simulink model "estimator_ekf_v02"  (Simulink 7.0)
settings: Solver=FixedStepDiscrete  StartTime=0  StopTime=0  FixedStep=1e-3  RelTol=1e-3
undefined symbols (not defined in the file): Ilf, Irf, l_fts, P0, Q, R, ROBOT, ts, X0
libraries: simulink x8
settings Model: Creator=raje_ra  LastModifiedBy=raje_ra  ExtModeAutoUpdateStatusClock=off
settings DebuggingCC: SignalInfNanChecking=error  CheckMatrixSingularityMsg=warning

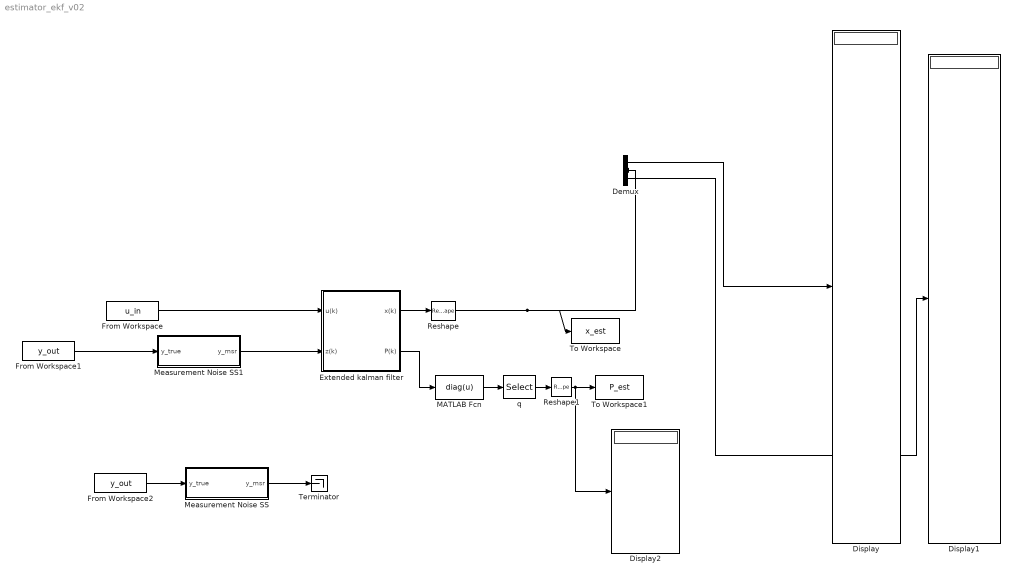
== system estimator_ekf_v02 ==
  Demux : Demux  Outputs=2
  Display : Display
  Display1 : Display
  Display2 : Display
  Extended kalman filter : Subsystem
  From Workspace : FromWorkspace  VariableName=u_in  SampleTime=0
  From Workspace1 : FromWorkspace  VariableName=y_out  SampleTime=0
  From Workspace2 : FromWorkspace  VariableName=y_out  SampleTime=0
  MATLAB Fcn : MATLABFcn  MATLABFcn=diag(u)  Output1D=off
  Measurement Noise SS : Subsystem
  Measurement Noise SS1 : Subsystem
  Reshape : Reshape
  Reshape1 : Reshape
  Terminator : Terminator
  To Workspace : ToWorkspace  VariableName=x_est  SampleTime=-1  SaveFormat=Structure With Time
  To Workspace1 : ToWorkspace  VariableName=P_est  SampleTime=-1  SaveFormat=Structure With Time
  q : Selector  InputPortWidth=62  IndexOptions=Index vector (dialog)  Indices=[1:6 32:37]  OutputSizes=1
  wires:
  Extended kalman filter/1(x(k)) -> Reshape/1
  From Workspace1/1 -> Measurement Noise SS1/1(y_true)
  From Workspace/1 -> Extended kalman filter/1(u(k))
  Reshape/1 -> To Workspace/1, Demux/1
  Measurement Noise SS/1(y_msr) -> Terminator/1
  From Workspace2/1 -> Measurement Noise SS/1(y_true)
  Measurement Noise SS1/1(y_msr) -> Extended kalman filter/2(z(k))
  Extended kalman filter/2(P(k)) -> MATLAB Fcn/1
  Demux/1 -> Display/1
  Demux/2 -> Display1/1
  MATLAB Fcn/1 -> q/1
  q/1 -> Reshape1/1
  Reshape1/1 -> To Workspace1/1, Display2/1

== system estimator_ekf_v02/Extended kalman filter ==
  u(k) : Inport  OutDataType=sfix(16)  OutScaling=2^0
  z(k) : Inport  Port=2  OutDataType=sfix(16)  OutScaling=2^0
  Unit Delay : UnitDelay  X0=X0  SampleTime=ts
  Unit Delay1 : UnitDelay  X0=P0  SampleTime=ts
  contact measurements : Subsystem
  corrector : Subsystem
  predictor : Subsystem
  x(k) : Outport  OutDataType=sfix(16)  OutScaling=2^0
  P(k) : Outport  Port=2  OutDataType=sfix(16)  OutScaling=2^0
  wires:
  u(k)/1 -> predictor/1(u(k)), corrector/2(u(k)), contact measurements/2(u_in(k))
  predictor/2(x_(k)-) -> corrector/4(x_(k)-)
  Unit Delay/1 -> predictor/2(x(k-1))
  corrector/1(x(k)) -> Unit Delay/1, x(k)/1  "x(k)"
  Unit Delay1/1 -> predictor/3(P(k-1))
  predictor/1(P_(k)-) -> corrector/3(P_(k)-)
  corrector/2(P(k)) -> Unit Delay1/1, P(k)/1
  z(k)/1 -> contact measurements/1(y(k))
  contact measurements/1(y) -> corrector/1(z(k))

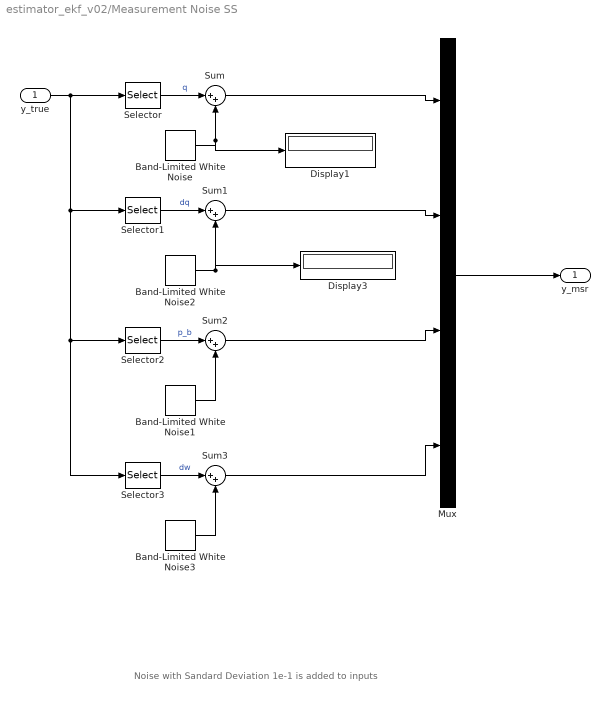
== system estimator_ekf_v02/Measurement Noise SS ==
  note: Noise with Sandard Deviation 1e-1 is added to inputs
  y_true : Inport  OutDataType=sfix(16)  OutScaling=2^0
  Band-Limited White Noise : simulink/Sources/Band-Limited White Noise  SystemSampleTime=-1  Cov=[1e-9]  Ts=ts  seed=[23341]
  Band-Limited White Noise1 : simulink/Sources/Band-Limited White Noise  SystemSampleTime=-1  Cov=[1e-8]  Ts=ts  seed=[23341]
  Band-Limited White Noise2 : simulink/Sources/Band-Limited White Noise  SystemSampleTime=-1  Cov=[1e-9]  Ts=ts  seed=[23341]
  Band-Limited White Noise3 : simulink/Sources/Band-Limited White Noise  SystemSampleTime=-1  Cov=[1e-9]  Ts=ts  seed=[23341]
  Display1 : Display
  Display3 : Display
  Mux : Mux
  Selector : Selector  InputPortWidth=m  IndexOptions=Index vector (dialog)  Indices=[1:25]  OutputSizes=1
  Selector1 : Selector  InputPortWidth=m  IndexOptions=Index vector (dialog)  Indices=[26:50]  OutputSizes=1
  Selector2 : Selector  InputPortWidth=m  IndexOptions=Index vector (dialog)  Indices=[51:53]  OutputSizes=1
  Selector3 : Selector  InputPortWidth=m  IndexOptions=Index vector (dialog)  Indices=[54:56]  OutputSizes=1
  Sum{,1..3} (4 alike) : Sum  Inputs=|++  OutDataType=sfix(16)  OutScaling=2^0
  y_msr : Outport
  wires:
  Band-Limited White Noise/1 -> Sum/2, Display1/1
  y_true/1 -> Selector/1, Selector1/1, Selector2/1, Selector3/1
  Selector/1 -> Sum/1  "q"
  Selector1/1 -> Sum1/1  "dq"
  Band-Limited White Noise2/1 -> Sum1/2, Display3/1
  Band-Limited White Noise1/1 -> Sum2/2
  Selector2/1 -> Sum2/1  "p_b"
  Band-Limited White Noise3/1 -> Sum3/2
  Selector3/1 -> Sum3/1  "dw"
  Sum/1 -> Mux/1
  Sum1/1 -> Mux/2
  Sum2/1 -> Mux/3
  Sum3/1 -> Mux/4
  Mux/1 -> y_msr/1

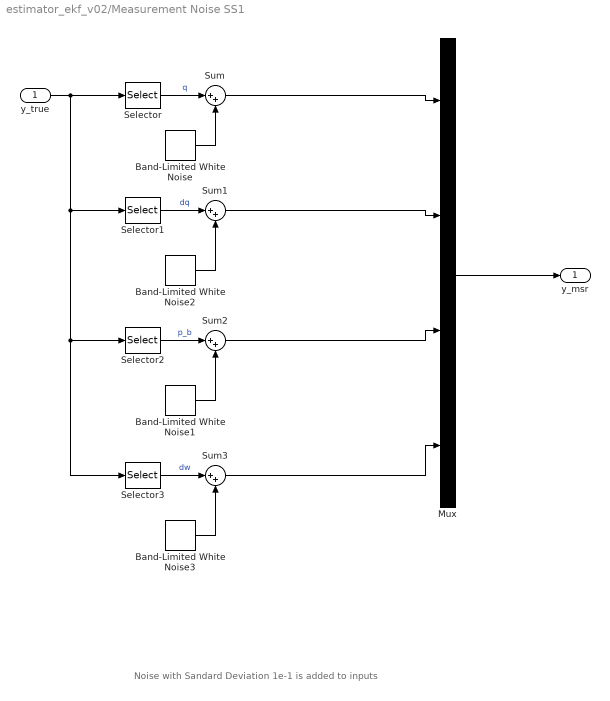
== system estimator_ekf_v02/Measurement Noise SS1 ==
  note: Noise with Sandard Deviation 1e-1 is added to inputs
  y_true : Inport  OutDataType=sfix(16)  OutScaling=2^0
  Band-Limited White Noise : simulink/Sources/Band-Limited White Noise  SystemSampleTime=-1  Cov=[1e-9]  Ts=ts  seed=[23341]
  Band-Limited White Noise1 : simulink/Sources/Band-Limited White Noise  SystemSampleTime=-1  Cov=[1e-5]  Ts=ts  seed=[23341]
  Band-Limited White Noise2 : simulink/Sources/Band-Limited White Noise  SystemSampleTime=-1  Cov=[1e-7]  Ts=ts  seed=[23341]
  Band-Limited White Noise3 : simulink/Sources/Band-Limited White Noise  SystemSampleTime=-1  Cov=[1e-7]  Ts=ts  seed=[23341]
  Mux : Mux
  Selector : Selector  InputPortWidth=m  IndexOptions=Index vector (dialog)  Indices=[1:25]  OutputSizes=1
  Selector1 : Selector  InputPortWidth=m  IndexOptions=Index vector (dialog)  Indices=[26:50]  OutputSizes=1
  Selector2 : Selector  InputPortWidth=m  IndexOptions=Index vector (dialog)  Indices=[51:53]  OutputSizes=1
  Selector3 : Selector  InputPortWidth=m  IndexOptions=Index vector (dialog)  Indices=[54:56]  OutputSizes=1
  Sum{,1..3} (4 alike) : Sum  Inputs=|++  OutDataType=sfix(16)  OutScaling=2^0
  y_msr : Outport
  wires:
  Mux/1 -> y_msr/1
  Sum3/1 -> Mux/4
  Sum2/1 -> Mux/3
  Sum1/1 -> Mux/2
  Sum/1 -> Mux/1
  Selector3/1 -> Sum3/1  "dw"
  Band-Limited White Noise3/1 -> Sum3/2
  Selector2/1 -> Sum2/1  "p_b"
  Band-Limited White Noise1/1 -> Sum2/2
  Band-Limited White Noise2/1 -> Sum1/2
  Selector1/1 -> Sum1/1  "dq"
  Selector/1 -> Sum/1  "q"
  y_true/1 -> Selector3/1, Selector2/1, Selector1/1, Selector/1
  Band-Limited White Noise/1 -> Sum/2

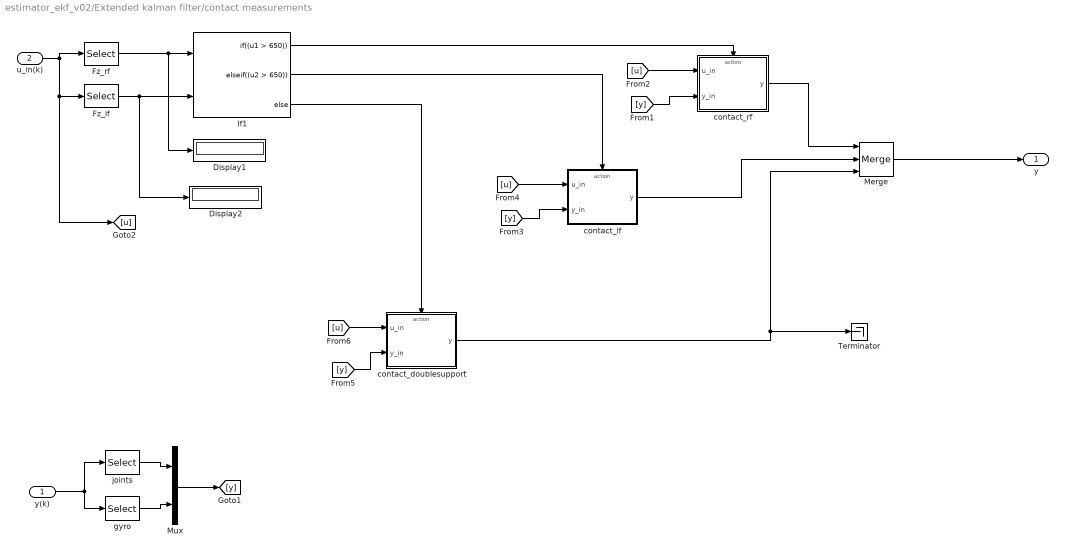
== system estimator_ekf_v02/Extended kalman filter/contact measurements ==
  y(k) : Inport
  u_in(k) : Inport  Port=2
  Display1 : Display
  Display2 : Display
  Fz_lf : Selector  InputPortWidth=37  IndexOptions=Index vector (dialog)  Indices=3  OutputSizes=1
  Fz_rf : Selector  InputPortWidth=37  IndexOptions=Index vector (dialog)  Indices=3  OutputSizes=1
  If1 : If  NumInputs=2  IfExpression=(u1 > 650)  ElseIfExpressions=(u2 > 650)
  Merge : Merge  Inputs=3
  Mux : Mux  Inputs=2
  Terminator : Terminator
  contact_doublesupport : Subsystem
  contact_lf : Subsystem
  contact_rf : Subsystem
  gyro : Selector  InputPortWidth=56  IndexOptions=Index vector (dialog)  Indices=[51:56]  OutputSizes=1
  joints : Selector  InputPortWidth=56  IndexOptions=Index vector (dialog)  Indices=1:50  OutputSizes=1
  y : Outport
  wires:
  Mux/1 -> [y]
  gyro/1 -> Mux/2
  joints/1 -> Mux/1
  contact_doublesupport/1(y) -> Merge/3, Terminator/1
  Merge/1 -> y/1
  contact_lf/1(y) -> Merge/2
  contact_rf/1(y) -> Merge/1
  If1/3 -> contact_doublesupport/Action
  If1/2 -> contact_lf/Action
  [y] -> contact_doublesupport/2(y_in)
  [u] -> contact_doublesupport/1(u_in)
  [y] -> contact_lf/2(y_in)
  [u] -> contact_lf/1(u_in)
  [y] -> contact_rf/2(y_in)
  [u] -> contact_rf/1(u_in)
  If1/1 -> contact_rf/Action
  u_in(k)/1 -> [u], Fz_lf/1, Fz_rf/1
  Fz_lf/1 -> Display2/1, If1/2
  Fz_rf/1 -> Display1/1, If1/1
  y(k)/1 -> gyro/1, joints/1

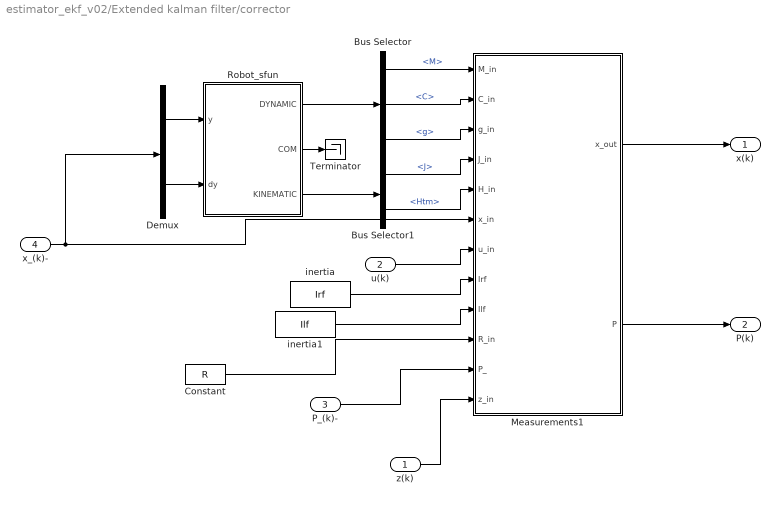
== system estimator_ekf_v02/Extended kalman filter/corrector ==
  z(k) : Inport  OutDataType=sfix(16)  OutScaling=2^0
  u(k) : Inport  Port=2  OutDataType=sfix(16)  OutScaling=2^0
  P_(k)- : Inport  Port=3  OutDataType=sfix(16)  OutScaling=2^0
  x_(k)- : Inport  Port=4  OutDataType=sfix(16)  OutScaling=2^0
  Bus Selector : BusSelector  OutputSignals=M,C,g
  Bus Selector1 : BusSelector  OutputSignals=J,Htm
  Constant : Constant  Value=R  OutDataType=sfix(16)  OutScaling=2^0
  Demux : Demux  Outputs=2
  Measurements1 : Stateflow chart
  Robot_sfun : Subsystem
  Terminator : Terminator
  inertia : Constant  Value=Irf  VectorParams1D=off  OutDataType=sfix(16)  OutScaling=2^0
  inertia1 : Constant  Value=Ilf  VectorParams1D=off  OutDataType=sfix(16)  OutScaling=2^0
  x(k) : Outport  OutDataType=sfix(16)  OutScaling=2^0
  P(k) : Outport  Port=2  OutDataType=sfix(16)  OutScaling=2^0
  wires:
  Robot_sfun/1(DYNAMIC) -> Bus Selector/1
  Bus Selector/1 -> Measurements1/1(M_in)  "<M>"
  Bus Selector/2 -> Measurements1/2(C_in)  "<C>"
  Bus Selector/3 -> Measurements1/3(g_in)  "<g>"
  Robot_sfun/3(KINEMATIC) -> Bus Selector1/1
  Bus Selector1/1 -> Measurements1/4(J_in)  "<J>"
  Bus Selector1/2 -> Measurements1/5(H_in)  "<Htm>"
  Demux/1 -> Robot_sfun/1(y)
  Demux/2 -> Robot_sfun/2(dy)
  Robot_sfun/2(COM) -> Terminator/1
  x_(k)-/1 -> Demux/1, Measurements1/6(x_in)
  Measurements1/1(x_out) -> x(k)/1
  u(k)/1 -> Measurements1/7(u_in)
  inertia/1 -> Measurements1/8(Irf)
  inertia1/1 -> Measurements1/9(Ilf)
  Constant/1 -> Measurements1/10(R_in)
  P_(k)-/1 -> Measurements1/11(P_)
  Measurements1/2(P) -> P(k)/1
  z(k)/1 -> Measurements1/12(z_in)

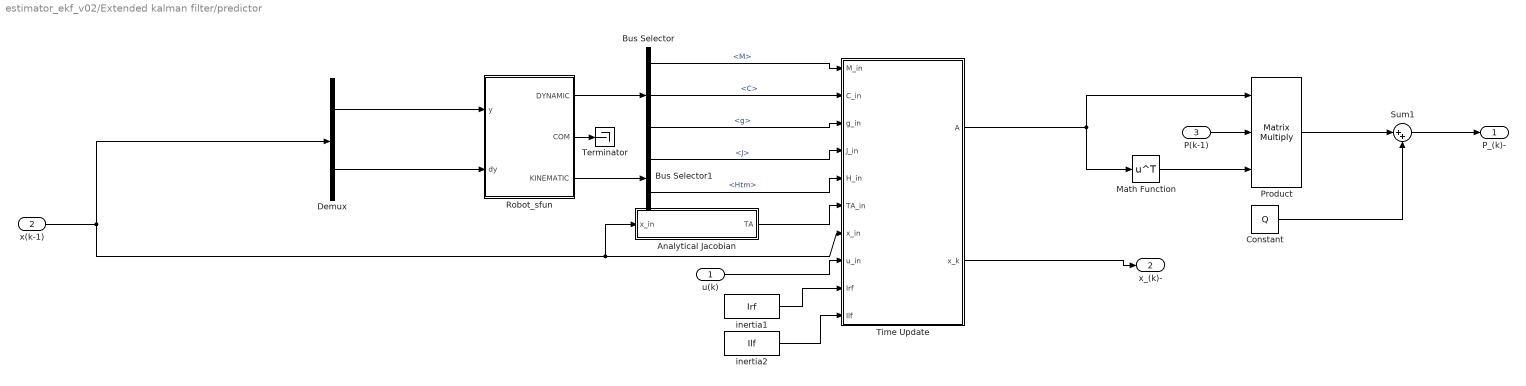
== system estimator_ekf_v02/Extended kalman filter/predictor ==
  u(k) : Inport  OutDataType=sfix(16)  OutScaling=2^0
  x(k-1) : Inport  Port=2  OutDataType=sfix(16)  OutScaling=2^0
  P(k-1) : Inport  Port=3  OutDataType=sfix(16)  OutScaling=2^0
  Analytical Jacobian : Stateflow chart
  Bus Selector : BusSelector  OutputSignals=M,C,g
  Bus Selector1 : BusSelector  OutputSignals=J,Htm
  Constant : Constant  Value=Q  OutDataType=sfix(16)  OutScaling=2^0
  Demux : Demux  Outputs=2
  Math Function : Math  Operator=transpose  OutDataType=sfix(16)  OutScaling=2^0  SaturateOnIntegerOverflow=on
  Product : Product  Inputs=3  Multiplication=Matrix(*)  OutDataType=sfix(16)  OutScaling=2^0  RndMeth=Zero
  Robot_sfun : Subsystem
  Sum1 : Sum  Inputs=|++  OutDataType=sfix(16)  OutScaling=2^0
  Terminator : Terminator
  Time Update : Stateflow chart
  inertia1 : Constant  Value=Irf  VectorParams1D=off  OutDataType=sfix(16)  OutScaling=2^0
  inertia2 : Constant  Value=Ilf  VectorParams1D=off  OutDataType=sfix(16)  OutScaling=2^0
  P_(k)- : Outport  OutDataType=sfix(16)  OutScaling=2^0
  x_(k)- : Outport  Port=2  OutDataType=sfix(16)  OutScaling=2^0
  wires:
  Robot_sfun/1(DYNAMIC) -> Bus Selector/1
  Bus Selector/1 -> Time Update/1(M_in)  "<M>"
  Bus Selector/2 -> Time Update/2(C_in)  "<C>"
  Bus Selector/3 -> Time Update/3(g_in)  "<g>"
  Robot_sfun/3(KINEMATIC) -> Bus Selector1/1
  Bus Selector1/1 -> Time Update/4(J_in)  "<J>"
  Bus Selector1/2 -> Time Update/5(H_in)  "<Htm>"
  x(k-1)/1 -> Analytical Jacobian/1(x_in), Time Update/7(x_in), Demux/1
  Demux/1 -> Robot_sfun/1(y)
  Demux/2 -> Robot_sfun/2(dy)
  Time Update/1(A) -> Math Function/1, Product/1
  Math Function/1 -> Product/3
  P(k-1)/1 -> Product/2
  Product/1 -> Sum1/1
  Constant/1 -> Sum1/2
  Sum1/1 -> P_(k)-/1
  Robot_sfun/2(COM) -> Terminator/1
  Analytical Jacobian/1(TA) -> Time Update/6(TA_in)
  u(k)/1 -> Time Update/8(u_in)
  inertia1/1 -> Time Update/9(Irf)
  inertia2/1 -> Time Update/10(Ilf)
  Time Update/2(x_k) -> x_(k)-/1

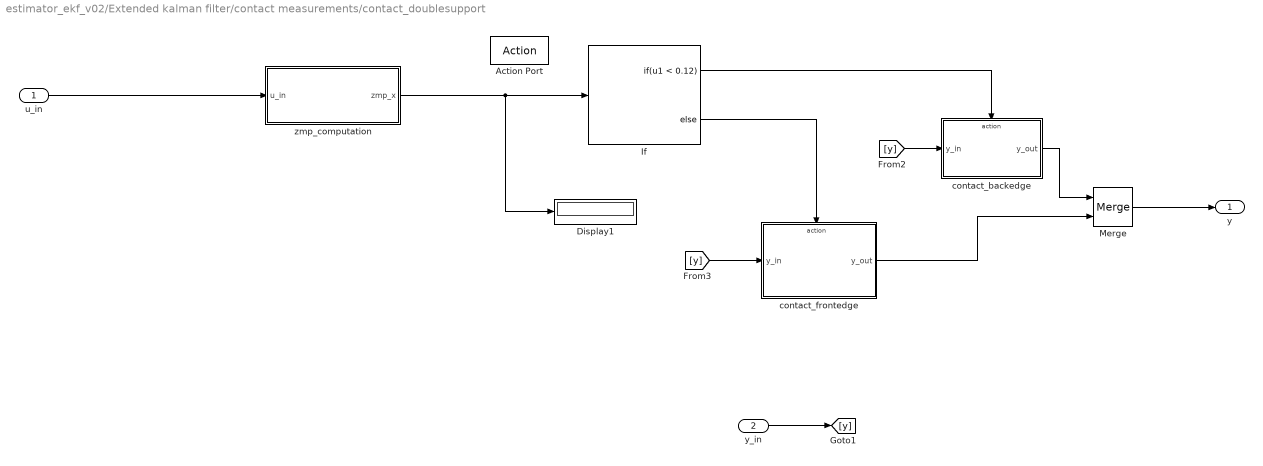
== system estimator_ekf_v02/Extended kalman filter/contact measurements/contact_doublesupport ==
  u_in : Inport
  y_in : Inport  Port=2
  Action Port : ActionPort  ActionType=else
  Display1 : Display
  If : If  IfExpression=u1 < 0.12
  Merge : Merge
  contact_backedge : Subsystem  TreatAsAtomicUnit=on
  contact_frontedge : Subsystem  TreatAsAtomicUnit=on
  zmp_computation : Subsystem
  y : Outport
  wires:
  u_in/1 -> zmp_computation/1(u_in)
  zmp_computation/1(zmp_x) -> Display1/1, If/1
  y_in/1 -> [y]
  Merge/1 -> y/1
  contact_frontedge/1(y_out) -> Merge/2
  contact_backedge/1(y_out) -> Merge/1
  [y] -> contact_frontedge/1(y_in)
  [y] -> contact_backedge/1(y_in)
  If/2 -> contact_frontedge/Action
  If/1 -> contact_backedge/Action

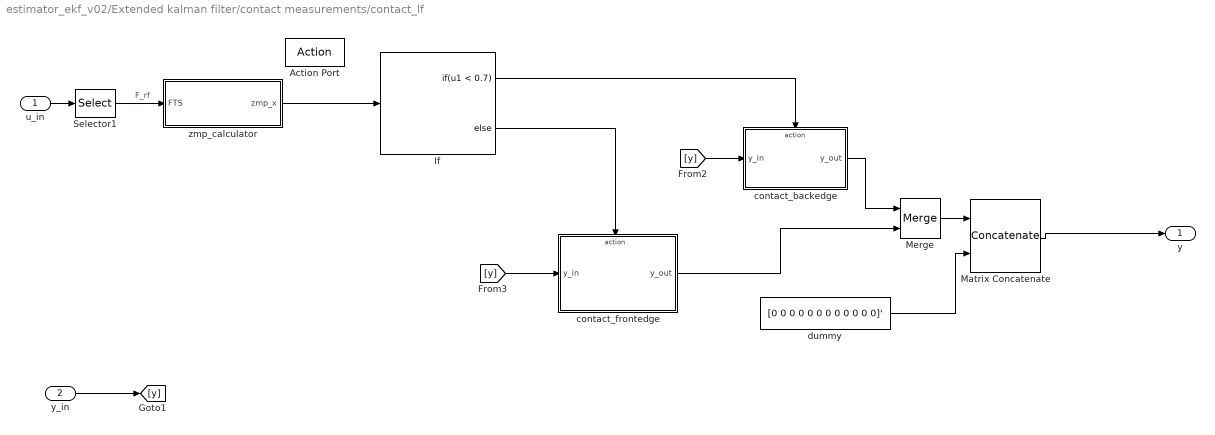
== system estimator_ekf_v02/Extended kalman filter/contact measurements/contact_lf ==
  u_in : Inport
  y_in : Inport  Port=2
  Action Port : ActionPort  ActionType=elseif
  If : If  IfExpression=u1 < 0.7
  Matrix Concatenate : Concatenate  Mode=Multidimensional array
  Merge : Merge
  Selector1 : Selector  InputPortWidth=37  IndexOptions=Index vector (dialog)  Indices=7:12  OutputSizes=1
  contact_backedge : Subsystem  TreatAsAtomicUnit=on
  contact_frontedge : Subsystem  TreatAsAtomicUnit=on
  dummy : Constant  Value=[0 0 0 0 0 0 0 0 0 0 0 0]'  VectorParams1D=off  OutDataType=sfix(16)  OutScaling=2^0
  zmp_calculator : Subsystem
  y : Outport
  wires:
  Matrix Concatenate/1 -> y/1
  dummy/1 -> Matrix Concatenate/2
  Merge/1 -> Matrix Concatenate/1
  If/1 -> contact_backedge/Action
  If/2 -> contact_frontedge/Action
  [y] -> contact_backedge/1(y_in)
  [y] -> contact_frontedge/1(y_in)
  contact_backedge/1(y_out) -> Merge/1
  contact_frontedge/1(y_out) -> Merge/2
  zmp_calculator/1(zmp_x) -> If/1
  Selector1/1 -> zmp_calculator/1(FTS)  "F_rf"
  u_in/1 -> Selector1/1
  y_in/1 -> [y]

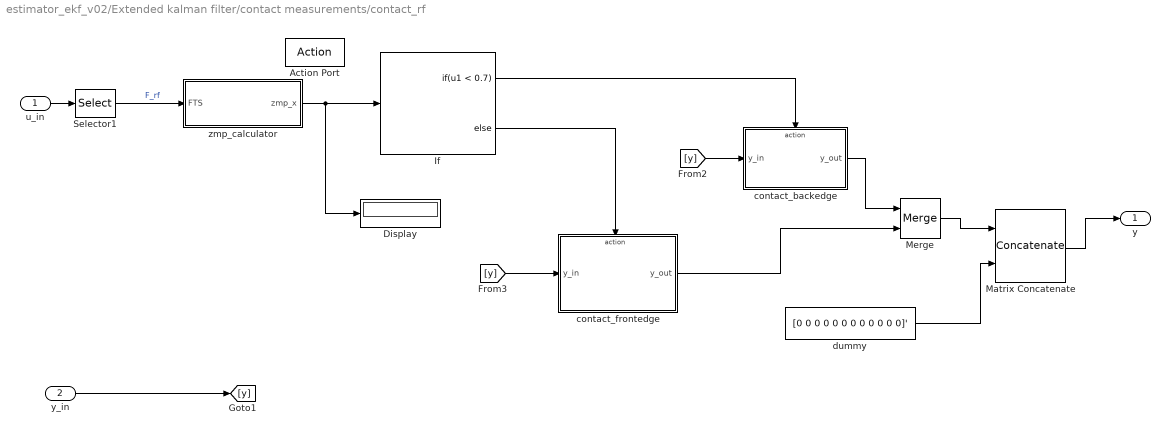
== system estimator_ekf_v02/Extended kalman filter/contact measurements/contact_rf ==
  u_in : Inport
  y_in : Inport  Port=2
  Action Port : ActionPort  ActionType=then
  Display : Display
  If : If  IfExpression=u1 < 0.7
  Matrix Concatenate : Concatenate  Mode=Multidimensional array
  Merge : Merge
  Selector1 : Selector  InputPortWidth=37  IndexOptions=Index vector (dialog)  Indices=1:6  OutputSizes=1
  contact_backedge : Subsystem  TreatAsAtomicUnit=on
  contact_frontedge : Subsystem  TreatAsAtomicUnit=on
  dummy : Constant  Value=[0 0 0 0 0 0 0 0 0 0 0 0]'  VectorParams1D=off  OutDataType=sfix(16)  OutScaling=2^0
  zmp_calculator : Subsystem
  y : Outport
  wires:
  Matrix Concatenate/1 -> y/1
  Merge/1 -> Matrix Concatenate/1
  dummy/1 -> Matrix Concatenate/2
  y_in/1 -> [y]
  u_in/1 -> Selector1/1
  Selector1/1 -> zmp_calculator/1(FTS)  "F_rf"
  zmp_calculator/1(zmp_x) -> Display/1, If/1
  contact_frontedge/1(y_out) -> Merge/2
  contact_backedge/1(y_out) -> Merge/1
  [y] -> contact_frontedge/1(y_in)
  [y] -> contact_backedge/1(y_in)
  If/2 -> contact_frontedge/Action
  If/1 -> contact_backedge/Action

== system estimator_ekf_v02/Extended kalman filter/corrector/Robot_sfun ==
  y : Inport
  dy : Inport  Port=2
  Bus Creator : BusCreator
  Bus Creator1 : BusCreator  Inputs=3
  Bus Creator2 : BusCreator  Inputs=3
  S-Function : S-Function  FunctionName=luca_dynamics_dy_sfun  Parameters=(size(ROBOT.csi,1)/6-1), size(ROBOT.csi,2), ROBOT.parent, ROBOT.tcp, ROBOT.g0, ROBOT.csi, ROBOT.com, ROBOT.Mass
  DYNAMIC : Outport
  COM : Outport  Port=2
  KINEMATIC : Outport  Port=3
  wires:
  y/1 -> S-Function/1
  dy/1 -> S-Function/2
  S-Function/1 -> Bus Creator/1  "M"
  S-Function/2 -> Bus Creator/2  "C"
  S-Function/3 -> Bus Creator/3  "g"
  S-Function/4 -> Bus Creator/4  "dM"
  S-Function/5 -> Bus Creator1/1  "x"
  S-Function/6 -> Bus Creator1/2  "J"
  S-Function/7 -> Bus Creator1/3  "dJ"
  S-Function/8 -> Bus Creator2/1  "Htm"
  S-Function/9 -> Bus Creator2/2  "J"
  S-Function/10 -> Bus Creator2/3  "dJ"
  Bus Creator/1 -> DYNAMIC/1
  Bus Creator1/1 -> COM/1
  Bus Creator2/1 -> KINEMATIC/1

== system estimator_ekf_v02/Extended kalman filter/predictor/Robot_sfun ==
  y : Inport
  dy : Inport  Port=2
  Bus Creator : BusCreator
  Bus Creator1 : BusCreator  Inputs=3
  Bus Creator2 : BusCreator  Inputs=3
  S-Function : S-Function  FunctionName=luca_dynamics_dy_sfun  Parameters=(size(ROBOT.csi,1)/6-1), size(ROBOT.csi,2), ROBOT.parent, ROBOT.tcp, ROBOT.g0, ROBOT.csi, ROBOT.com, ROBOT.Mass
  DYNAMIC : Outport
  COM : Outport  Port=2
  KINEMATIC : Outport  Port=3
  wires:
  Bus Creator2/1 -> KINEMATIC/1
  Bus Creator1/1 -> COM/1
  Bus Creator/1 -> DYNAMIC/1
  S-Function/10 -> Bus Creator2/3  "dJ"
  S-Function/9 -> Bus Creator2/2  "J"
  S-Function/8 -> Bus Creator2/1  "Htm"
  S-Function/7 -> Bus Creator1/3  "dJ"
  S-Function/6 -> Bus Creator1/2  "J"
  S-Function/5 -> Bus Creator1/1  "x"
  S-Function/4 -> Bus Creator/4  "dM"
  S-Function/3 -> Bus Creator/3  "g"
  S-Function/2 -> Bus Creator/2  "C"
  S-Function/1 -> Bus Creator/1  "M"
  dy/1 -> S-Function/2
  y/1 -> S-Function/1

== system estimator_ekf_v02/Extended kalman filter/contact measurements/contact_doublesupport/contact_backedge ==
  y_in : Inport  OutDataType=sfix(16)  OutScaling=2^0
  Action Port : ActionPort  ActionType=then
  Matrix Concatenate : Concatenate  NumInputs=4  Mode=Multidimensional array
  V_feet : Constant  Value=[0 0 0 0 0 0 0 0 0 0 0 0]'  VectorParams1D=off  OutDataType=sfix(16)  OutScaling=2^0
  lf_contact_CD : Constant  Value="[-0.059999942250943   0.065450013201346  -0.000099999469068  -0.059999926220207   0.160450013201344  -0.000099995026751]'"  VectorParams1D=off  OutDataType=sfix(16)  OutScaling=2^0
  rf_contact_CD : Constant  Value="[-0.059999991262275  -0.160449976611997  -0.000099795625568  -0.059999972932080  -0.065449976612284  -0.000099562918613]'"  VectorParams1D=off  OutDataType=sfix(16)  OutScaling=2^0
  y_out : Outport  OutDataType=sfix(16)  OutScaling=2^0
  wires:
  V_feet/1 -> Matrix Concatenate/4
  lf_contact_CD/1 -> Matrix Concatenate/3
  rf_contact_CD/1 -> Matrix Concatenate/2
  Matrix Concatenate/1 -> y_out/1
  y_in/1 -> Matrix Concatenate/1

== system estimator_ekf_v02/Extended kalman filter/contact measurements/contact_doublesupport/contact_frontedge ==
  y_in : Inport  OutDataType=sfix(16)  OutScaling=2^0
  Action Port : ActionPort  ActionType=else
  Matrix Concatenate : Concatenate  NumInputs=4  Mode=Multidimensional array
  V_feet : Constant  Value=[0 0 0 0 0 0 0 0 0 0 0 0]'  VectorParams1D=off  OutDataType=sfix(16)  OutScaling=2^0
  lf_contact_AB : Constant  Value="[0.130000073779718   0.160449981139864  -0.000099828958185   0.130000057748982   0.065449981139865  -0.000099833400502]'"  VectorParams1D=off  OutDataType=sfix(16)  OutScaling=2^0
  rf_contact_AB : Constant  Value="[0.130000027067808  -0.065450013272176  -0.000099766533171   0.130000008737612  -0.160450013271890  -0.000099999240125]'"  VectorParams1D=off  OutDataType=sfix(16)  OutScaling=2^0
  y_out : Outport  OutDataType=sfix(16)  OutScaling=2^0
  wires:
  V_feet/1 -> Matrix Concatenate/4
  lf_contact_AB/1 -> Matrix Concatenate/3
  rf_contact_AB/1 -> Matrix Concatenate/2
  Matrix Concatenate/1 -> y_out/1
  y_in/1 -> Matrix Concatenate/1

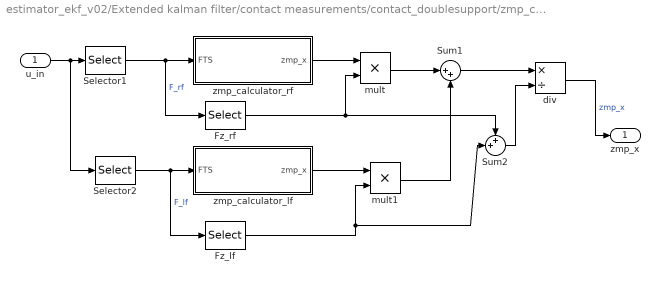
== system estimator_ekf_v02/Extended kalman filter/contact measurements/contact_doublesupport/zmp_computation ==
  u_in : Inport
  Fz_lf : Selector  InputPortWidth=6  IndexOptions=Index vector (dialog)  Indices=3  OutputSizes=1
  Fz_rf : Selector  InputPortWidth=6  IndexOptions=Index vector (dialog)  Indices=3  OutputSizes=1
  Selector1 : Selector  InputPortWidth=37  IndexOptions=Index vector (dialog)  Indices=1:6  OutputSizes=1
  Selector2 : Selector  InputPortWidth=37  IndexOptions=Index vector (dialog)  Indices=7:12  OutputSizes=1
  Sum1 : Sum  Inputs=|++  OutDataType=sfix(16)  OutScaling=2^0
  Sum2 : Sum  Inputs=++|  OutDataType=sfix(16)  OutScaling=2^0
  div : Product  Inputs=*/  OutDataType=sfix(16)  OutScaling=2^-10
  mult : Product  Inputs=**  OutDataType=sfix(16)  OutScaling=2^-10
  mult1 : Product  Inputs=**  OutDataType=sfix(16)  OutScaling=2^-10
  zmp_calculator_lf : Subsystem
  zmp_calculator_rf : Subsystem
  zmp_x : Outport
  wires:
  div/1 -> zmp_x/1  "zmp_x"
  Sum2/1 -> div/2
  Sum1/1 -> div/1
  mult1/1 -> Sum1/2
  zmp_calculator_lf/1(zmp_x) -> mult1/1
  mult/1 -> Sum1/1
  zmp_calculator_rf/1(zmp_x) -> mult/1
  Fz_rf/1 -> Sum2/1, mult/2
  Fz_lf/1 -> Sum2/2, mult1/2
  Selector2/1 -> Fz_lf/1, zmp_calculator_lf/1(FTS)  "F_lf"
  u_in/1 -> Selector2/1, Selector1/1
  Selector1/1 -> Fz_rf/1, zmp_calculator_rf/1(FTS)  "F_rf"

== system estimator_ekf_v02/Extended kalman filter/contact measurements/contact_lf/contact_backedge ==
  y_in : Inport  OutDataType=sfix(16)  OutScaling=2^0
  Action Port : ActionPort  ActionType=then
  Matrix Concatenate : Concatenate  NumInputs=3  Mode=Multidimensional array
  V_lf : Constant  Value=[0 0 0 0 0 0]'  VectorParams1D=off  OutDataType=sfix(16)  OutScaling=2^0
  lf_contact_CD : Constant  Value="[-0.059999942250943   0.065450013201346  -0.000099999469068  -0.059999926220207   0.160450013201344  -0.000099995026751]'"  VectorParams1D=off  OutDataType=sfix(16)  OutScaling=2^0
  y_out : Outport  OutDataType=sfix(16)  OutScaling=2^0
  wires:
  lf_contact_CD/1 -> Matrix Concatenate/2
  y_in/1 -> Matrix Concatenate/1
  Matrix Concatenate/1 -> y_out/1
  V_lf/1 -> Matrix Concatenate/3

== system estimator_ekf_v02/Extended kalman filter/contact measurements/contact_lf/contact_frontedge ==
  y_in : Inport  OutDataType=sfix(16)  OutScaling=2^0
  Action Port : ActionPort  ActionType=else
  Matrix Concatenate : Concatenate  NumInputs=3  Mode=Multidimensional array
  V_lf : Constant  Value=[0 0 0 0 0 0]'  VectorParams1D=off  OutDataType=sfix(16)  OutScaling=2^0
  lf_contact_AB : Constant  Value="[0.130000073779718   0.160449981139864  -0.000099828958185   0.130000057748982   0.065449981139865  -0.000099833400502]'"  VectorParams1D=off  OutDataType=sfix(16)  OutScaling=2^0
  y_out : Outport  OutDataType=sfix(16)  OutScaling=2^0
  wires:
  V_lf/1 -> Matrix Concatenate/3
  lf_contact_AB/1 -> Matrix Concatenate/2
  y_in/1 -> Matrix Concatenate/1
  Matrix Concatenate/1 -> y_out/1

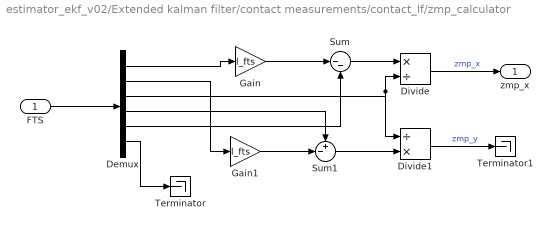
== system estimator_ekf_v02/Extended kalman filter/contact measurements/contact_lf/zmp_calculator ==
  FTS : Inport
  Demux : Demux  Outputs=6
  Divide : Product  Inputs=*/  OutDataType=sfix(16)  OutScaling=2^-10
  Divide1 : Product  Inputs=/*  OutDataType=sfix(16)  OutScaling=2^-10
  Gain : Gain  Gain=l_fts  ParameterDataType=sfix(16)  ParameterScaling=2^0  OutDataType=sfix(16)  OutScaling=2^0
  Gain1 : Gain  Gain=l_fts  ParameterDataType=sfix(16)  ParameterScaling=2^0  OutDataType=sfix(16)  OutScaling=2^0
  Sum : Sum  Inputs=|--  OutDataType=sfix(16)  OutScaling=2^0
  Sum1 : Sum  Inputs=+-|  OutDataType=sfix(16)  OutScaling=2^0
  Terminator : Terminator
  Terminator1 : Terminator
  zmp_x : Outport
  wires:
  Demux/1 -> Gain/1
  Gain/1 -> Sum/1
  Demux/5 -> Sum/2
  Sum/1 -> Divide/1
  Demux/3 -> Divide/2, Divide1/1
  Demux/2 -> Gain1/1
  Gain1/1 -> Sum1/2
  Demux/4 -> Sum1/1
  Sum1/1 -> Divide1/2
  Demux/6 -> Terminator/1
  Divide1/1 -> Terminator1/1  "zmp_y"
  Divide/1 -> zmp_x/1  "zmp_x"
  FTS/1 -> Demux/1

== system estimator_ekf_v02/Extended kalman filter/contact measurements/contact_rf/contact_backedge ==
  y_in : Inport  OutDataType=sfix(16)  OutScaling=2^0
  Action Port : ActionPort  ActionType=then
  Matrix Concatenate : Concatenate  NumInputs=3  Mode=Multidimensional array
  V_rf : Constant  Value=[0 0 0 0 0 0]'  VectorParams1D=off  OutDataType=sfix(16)  OutScaling=2^0
  rf_contact_CD : Constant  Value="[-0.059999991262275  -0.160449976611997  -0.000099795625568  -0.059999972932080  -0.065449976612284  -0.000099562918613]'"  VectorParams1D=off  OutDataType=sfix(16)  OutScaling=2^0
  y_out : Outport  OutDataType=sfix(16)  OutScaling=2^0
  wires:
  V_rf/1 -> Matrix Concatenate/3
  rf_contact_CD/1 -> Matrix Concatenate/2
  Matrix Concatenate/1 -> y_out/1
  y_in/1 -> Matrix Concatenate/1

== system estimator_ekf_v02/Extended kalman filter/contact measurements/contact_rf/contact_frontedge ==
  y_in : Inport  OutDataType=sfix(16)  OutScaling=2^0
  Action Port : ActionPort  ActionType=else
  Matrix Concatenate : Concatenate  NumInputs=3  Mode=Multidimensional array
  V_rf : Constant  Value=[0 0 0 0 0 0]'  VectorParams1D=off  OutDataType=sfix(16)  OutScaling=2^0
  rf_contact_AB : Constant  Value="[0.130000027067808  -0.065450013272176  -0.000099766533171   0.130000008737612  -0.160450013271890  -0.000099999240125]'"  VectorParams1D=off  OutDataType=sfix(16)  OutScaling=2^0
  y_out : Outport  OutDataType=sfix(16)  OutScaling=2^0
  wires:
  V_rf/1 -> Matrix Concatenate/3
  rf_contact_AB/1 -> Matrix Concatenate/2
  Matrix Concatenate/1 -> y_out/1
  y_in/1 -> Matrix Concatenate/1

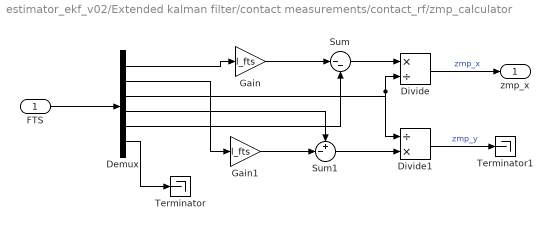
== system estimator_ekf_v02/Extended kalman filter/contact measurements/contact_rf/zmp_calculator ==
  FTS : Inport
  Demux : Demux  Outputs=6
  Divide : Product  Inputs=*/  OutDataType=sfix(16)  OutScaling=2^-10
  Divide1 : Product  Inputs=/*  OutDataType=sfix(16)  OutScaling=2^-10
  Gain : Gain  Gain=l_fts  ParameterDataType=sfix(16)  ParameterScaling=2^0  OutDataType=sfix(16)  OutScaling=2^0
  Gain1 : Gain  Gain=l_fts  ParameterDataType=sfix(16)  ParameterScaling=2^0  OutDataType=sfix(16)  OutScaling=2^0
  Sum : Sum  Inputs=|--  OutDataType=sfix(16)  OutScaling=2^0
  Sum1 : Sum  Inputs=+-|  OutDataType=sfix(16)  OutScaling=2^0
  Terminator : Terminator
  Terminator1 : Terminator
  zmp_x : Outport
  wires:
  FTS/1 -> Demux/1
  Divide/1 -> zmp_x/1  "zmp_x"
  Divide1/1 -> Terminator1/1  "zmp_y"
  Demux/6 -> Terminator/1
  Sum1/1 -> Divide1/2
  Demux/4 -> Sum1/1
  Gain1/1 -> Sum1/2
  Demux/2 -> Gain1/1
  Demux/3 -> Divide1/1, Divide/2
  Sum/1 -> Divide/1
  Demux/5 -> Sum/2
  Gain/1 -> Sum/1
  Demux/1 -> Gain/1

== system estimator_ekf_v02/Extended kalman filter/contact measurements/contact_doublesupport/zmp_computation/zmp_calculator_lf ==
  FTS : Inport
  Demux : Demux  Outputs=6
  Divide : Product  Inputs=*/  OutDataType=sfix(16)  OutScaling=2^-10
  Divide1 : Product  Inputs=/*  OutDataType=sfix(16)  OutScaling=2^-10
  Gain : Gain  Gain=l_fts  ParameterDataType=sfix(16)  ParameterScaling=2^0  OutDataType=sfix(16)  OutScaling=2^0
  Gain1 : Gain  Gain=l_fts  ParameterDataType=sfix(16)  ParameterScaling=2^0  OutDataType=sfix(16)  OutScaling=2^0
  Sum : Sum  Inputs=|--  OutDataType=sfix(16)  OutScaling=2^0
  Sum1 : Sum  Inputs=+-|  OutDataType=sfix(16)  OutScaling=2^0
  Terminator : Terminator
  Terminator1 : Terminator
  zmp_x : Outport
  wires:
  Demux/1 -> Gain/1
  Gain/1 -> Sum/1
  Demux/5 -> Sum/2
  Sum/1 -> Divide/1
  Demux/3 -> Divide/2, Divide1/1
  Demux/2 -> Gain1/1
  Gain1/1 -> Sum1/2
  Demux/4 -> Sum1/1
  Sum1/1 -> Divide1/2
  Demux/6 -> Terminator/1
  Divide1/1 -> Terminator1/1  "zmp_y"
  Divide/1 -> zmp_x/1  "zmp_x"
  FTS/1 -> Demux/1

== system estimator_ekf_v02/Extended kalman filter/contact measurements/contact_doublesupport/zmp_computation/zmp_calculator_rf ==
  FTS : Inport
  Demux : Demux  Outputs=6
  Divide : Product  Inputs=*/  OutDataType=sfix(16)  OutScaling=2^-10
  Divide1 : Product  Inputs=/*  OutDataType=sfix(16)  OutScaling=2^-10
  Gain : Gain  Gain=l_fts  ParameterDataType=sfix(16)  ParameterScaling=2^0  OutDataType=sfix(16)  OutScaling=2^0
  Gain1 : Gain  Gain=l_fts  ParameterDataType=sfix(16)  ParameterScaling=2^0  OutDataType=sfix(16)  OutScaling=2^0
  Sum : Sum  Inputs=|--  OutDataType=sfix(16)  OutScaling=2^0
  Sum1 : Sum  Inputs=+-|  OutDataType=sfix(16)  OutScaling=2^0
  Terminator : Terminator
  Terminator1 : Terminator
  zmp_x : Outport
  wires:
  FTS/1 -> Demux/1
  Divide/1 -> zmp_x/1  "zmp_x"
  Divide1/1 -> Terminator1/1  "zmp_y"
  Demux/6 -> Terminator/1
  Sum1/1 -> Divide1/2
  Demux/4 -> Sum1/1
  Gain1/1 -> Sum1/2
  Demux/2 -> Gain1/1
  Demux/3 -> Divide1/1, Divide/2
  Sum/1 -> Divide/1
  Demux/5 -> Sum/2
  Gain/1 -> Sum/1
  Demux/1 -> Gain/1

== matlab function Extended kalman filter/predictor/Analytical Jacobian ==
  data: TA output inherited; x_in input inherited
function TA = fcn(x_in)
% This block supports the Embedded MATLAB subset.
% See the help menu for details. 
% state - [ position ; velocity ]
% x_in  - [   1:31   ;   32:62  ]
ox = x_in(4);
oy = x_in(5);
% Transformation for Angular velocities to angular rates of floating base 
% on instantaneous frame of reference. x-y-z rotations.
%%{
T = [1      0           sin(oy);...
     0 cos(ox) -cos(oy)*sin(ox);...
     0 sin(ox)  cos(oy)*cos(ox)];


dTx = [0,         0,                0 ;...
       0,  -sin(ox),  -cos(oy)*cos(ox);...
       0,   cos(ox),  -cos(oy)*sin(ox)];
dTy = [0,         0,           cos(oy);...
       0,         0,   sin(oy)*sin(ox);...
       0,         0,  -sin(oy)*cos(ox)];
%%}

%{
T = [1      0   -sin(oy);...
     0  cos(ox)  cos(oy)*sin(ox);...
     0 -sin(ox)  cos(oy)*cos(ox)];
 
%T_A = [eye(3,6);zeros(3),T];

dTx = [0         0                0 ;
       0   -sin(ox)  cos(oy)*cos(ox);
       0   -cos(ox) -cos(oy)*sin(ox)];
dTy = [0       0        -cos(oy);
       0       0        -sin(oy)*sin(ox);
       0       0        -sin(oy)*cos(ox)];
%}

%TA = [ T_A; zeros(3*6,6); [zeros(3,6); [zeros(3) dTx]] ; [zeros(3,6); [zeros(3) dTy]]; zeros(57*6,6) ];

TA = [ T; dTx;dTy;zeros(3,3)];

== matlab function Extended kalman filter/predictor/Time Update ==
  data: A output inherited; M_in input inherited; x_k output inherited; C_in input inherited; g_in input inherited; J_in input inherited; H_in input inherited; TA_in input inherited; x_in input inherited; u_in input inherited; Irf input inherited; Ilf input inherited
function [A,x_k]= fcn(M_in,C_in,g_in,J_in,H_in,TA_in,x_in,u_in,Irf,Ilf)
% This block supports the Embedded MATLAB subset.
% See the help menu for details. 

dt = 1e-3;
dof = 31;
ind4 = -3:0;
ind6 = -5:0;

% Dynamic parameters
M = M_in(1:dof,:);
C = C_in(1:dof,:);
grav = g_in(1:dof);

invM = M \ eye(dof,dof);
% Kinematics
% tcp = 1 - Right Foot ; 2 - Left Foot ; 3 - Right Hand ; 4 - Left Hand ;
%       5 - Floating Base

Jrf = J_in(1*6+ind6,:);
Jlf = J_in(2*6+ind6,:);

Hrf = H_in(1*4+ind4,:);
Rrf = Hrf(1:3,1:3);
prf = Skew(Hrf(1:3,4));

Hlf = H_in(2*4+ind4,:);
Rlf = Hlf(1:3,1:3);
plf = Skew(Hlf(1:3,4));

Hfb = H_in(5*4+ind4,:);
Rfb = Hfb(1:3,1:3);

% state - [ position ; velocity ]
% x_in  - [   1:31   ;   32:62  ]
%q = x_in(1:dof);
dq = x_in(dof+(1:dof));

% inputs - [FTS_RF ; FTS _LF ; TRQ_JOINT]
% u_in   - [  1:6  ;   7:12  ;  13:37   ]
Frf = u_in(1*6+ind6,:);
Flf = u_in(2*6+ind6,:);
tau = [zeros(6,1); u_in(13:37)];

% Transformation for Angular velocities to angular rates of floating base 
% on instantaneous frame of reference. x-y-z rotations.
TA = TA_in(1:3,:);
invTA = TA \ eye(3,3);
% Transformation from body to spacial frame:
%Adfb = Adjoint(Hfb);
Adrf = Adjoint(Hrf);
Adlf = Adjoint(Hlf);

invAdrf = InvAdjoint(Hrf);
invAdlf = InvAdjoint(Hlf);

% Transformation for the velocites of floating base
vfb = dq(1:3);
wfb = dq(4:6);

dp = Rfb * vfb;
do = invTA * (Rfb*wfb);

vel = [dp; do; dq(7:31)];

%vel = [Vfb_s; dq(7:31)];%~~~~~~~ First Attempt

gacc = [ 0 0 -9.81 0 0 0]';
% errrf = Irf * (Adrf\gacc) ;
% errlf = Ilf * (Adlf\gacc);
errrf = Irf * invAdrf * gacc ;
errlf = Ilf * invAdlf * gacc ;


% Computation of accelerations
%acc = M \ (-C*dq - grav + tau + Jrf'*Adrf'*Frf + Jlf'*Adlf'*Flf - Jrf'*errrf - Jlf'*errlf);
acc = invM * (-C*dq - grav + tau + Jrf'*Adrf'*Frf + Jlf'*Adlf'*Flf - Jrf'*errrf - Jlf'*errlf);
x_dot = [vel;acc];   

% Computing second order derivative terms for base
% p - position of floating base o-orientation of floating base

x_k = x_in + dt*x_dot ;


% Computation of Jacobian for velocities of Floating base

dqdx = [zeros(25,37),eye(25)];                               %%%%%%%%%%%%%%%%

% Compute the Jacobian of acceleration terms(forward dynamics):
dpdx = zeros(3,2*dof);
dodx = zeros(3,2*dof);

dacc = zeros(dof,2*dof);
for i = 1:62
    dM   = M_in(i*dof+(1:dof),:);
    dC   = C_in(i*dof+(1:dof),:);
    dg   = g_in(i*dof+(1:dof));
    dJrf = J_in(i*30+(1*6+ind6),:);
    dJlf = J_in(i*30+(2*6+ind6),:);
    
    dHrf = H_in(i*20+(1*4+ind4),:);
    dRrf = dHrf(1:3,1:3);
    dprf = Skew(dHrf(1:3,4));
    dAdrf   = [ dRrf dprf*Rrf+prf*dRrf ; zeros(3) dRrf ];
    
    dHlf = H_in(i*20+(2*4+ind4),:); 
    dRlf = dHlf(1:3,1:3);
    dplf = Skew(dHlf(1:3,4));
    dAdlf   = [ dRlf dplf*Rlf+plf*dRlf ; zeros(3) dRlf ];
    
    dHfb  = H_in(i*20+(5*4+ind4),:); 
    dRfb  = dHfb( 1:3, 1:3);
 
    dpdx(:,i) = dRfb*vfb;
    %dodx(:,i) = TA \ ( dRfb*wfb) ;
    dodx(:,i) = invTA * ( dRfb*wfb) ;

    if i > 3 && i < 6
        
    dTA   = TA_in((i-3)*3+(1:3),:);
    % dodx(:,i) = TA\ (-dTA*do );
    dodx(:,i) = dodx(:,i) + invTA * (-dTA*do );
    
    end 

%     dacc(:,i)   = M \ (-dM*acc +(-dC*dq - dg + dJrf'*Adrf'*Frf + Jrf'*dAdrf'*Frf...
%                                              + dJlf'*Adlf'*Flf + Jlf'*dAdlf'*Flf...
%                                              - ( dJrf'*Irf*(Adrf\gacc) + Jrf'*(-Adrf\(dAdrf*(Adrf\gacc))) ) ...
%                                              - ( dJlf'*Ilf*(Adlf\gacc) + Jlf'*(-Adlf\(dAdlf*(Adlf\gacc))) ) ));
      dacc(:,i)   = invM * (-dM*acc +(-dC*dq - dg + dJrf'*Adrf'*Frf + Jrf'*dAdrf'*Frf...
                                              + dJlf'*Adlf'*Flf + Jlf'*dAdlf'*Flf...
                                              - ( dJrf'*Irf* (invAdrf * gacc) + Jrf'*(-invAdrf *(dAdrf*(invAdrf * gacc))) ) ...
                                              - ( dJlf'*Ilf* (invAdlf * gacc) + Jlf'*(-invAdlf *(dAdlf*(invAdlf * gacc))) ) ));
    
    if i > dof
        if i <= dof+3
            dpdx(:,i) = dpdx(:,i) + Rfb(:,i-dof);         
        elseif i<= dof+6
            %dodx(:,i) = dodx(:,i) + TA\Rfb(:,i-(dof+3)); 
            dodx(:,i) = dodx(:,i) + invTA * Rfb(:,i-(dof+3)); 
        end
        %dacc(:,i) = dacc(:,i) + M \ (- C(:,i-31));
        dacc(:,i) = dacc(:,i) + invM * (- C(:,i-31));

    end
end

dvel = [ dpdx ; dodx ; dqdx ];

A = eye(62) + dt * [dvel;dacc] ;

== matlab function Extended kalman filter/corrector/Measurements1 ==
  data: M_in input inherited; x_out output inherited; C_in input inherited; g_in input inherited; J_in input inherited; H_in input inherited; x_in input inherited; u_in input inherited; Irf input inherited; Ilf input inherited; R_in input inherited; P_ input inherited; P output inherited; z_in input inherited
function [x_out,P]= fcn(M_in,C_in,g_in,J_in,H_in,x_in,u_in,Irf,Ilf,R_in,P_,z_in)
% This block supports the Embedded MATLAB subset.
% See the help menu for details. 

dof = 31;
ind4 = -3:0;
ind6 = -5:0;

% Dynamic parameters
M = M_in(1:dof,:);
C = C_in(1:dof,:);
grav = g_in(1:dof);

invM = M \ eye(dof,dof);

% Kinematics
% tcp = 1 - Right Foot ; 2 - Left Foot ; 3 - Right Hand ; 4 - Left Hand ;
%       5 - Floating Base

Jrf = J_in(1*6+ind6,:);
Jlf = J_in(2*6+ind6,:);

Hrf = H_in(1*4+ind4,:);
Rrf = Hrf(1:3,1:3);
prf = Skew(Hrf(1:3,4));

Hlf = H_in(2*4+ind4,:);
Rlf = Hlf(1:3,1:3);
plf = Skew(Hlf(1:3,4));

Hfb = H_in(5*4+ind4,:);
Rfb = Hfb(1:3,1:3);


Adrf = Adjoint(Hrf);
Adlf = Adjoint(Hlf);

invAdrf = InvAdjoint(Hrf);
invAdlf = InvAdjoint(Hlf);

% state - [ position ; velocity ]
% x_in  - [   1:31   ;   32:62  ]
q = x_in(1:dof);
dq = x_in(dof+(1:dof));
omega = dq(4:6);

% inputs - [FTS_RF ; FTS _LF ; TRQ_JOINT]
% u_in   - [  1:6  ;   7:12  ;  13:37   ]
Frf = u_in(1*6+ind6,:);
Flf = u_in(2*6+ind6,:);
tau = [zeros(6,1); u_in(13:37)];

% Transformation for Angular velocities to angular rates of floating base 
% on instantaneous frame of reference. x-y-z rotations.
%TA = TA_in(1*6+ind6,:);

% Gyroscopic measurements
%gyro = Rfb'*( TA(4:6,4:6) \ (Rfb*omega) ); % ~~~~~~~~~~~~~~~~~~~~~~~~Not sure weather this is correct ????????????
 gyro = omega;                                          % Should the gyroscope be necessarily rotated ???

% Inertia correction

gacc = [ 0 0 -9.81 0 0 0]';
errrf = Irf * invAdrf * gacc ;
errlf = Ilf * invAdlf * gacc ;


% Computation of accelerations
acc = invM * (-C*dq - grav + tau + Jrf'*Adrf'*Frf + Jlf'*Adlf'*Flf - Jrf'*errrf - Jlf'*errlf);

% Gravity compensation for IMU
imu_bias = [ 0.005 0 0]';
imu = acc(1:3) + Rfb'*[0 0 9.81]'+imu_bias;

%Internal sensors
jnt = [q(7:31);dq(7:31)];

% Velocity measurements for foot contact
%v_rf = Jr*v; 
%v_lf = Jl*v;
%msr_vcont = [v_rf;v_lf];

% Position of the contact points
% Contact Model:
%        y       b---------c
%        |       |      .o |
%    x_ _|       a---------d
%
% CD --> AB === Fx: 20 --> -20
% AB --> CD === Fx: -20 --> 20

contact_AB = [ 0.13 0.0475 0 1 0.13 -0.0475 0 1]';
contact_CD = [ -0.06 -0.0475 0 1 -0.06 0.0475 0 1]';

% zmp computation
zmprf_x = ( -Frf(5) -0.1189 * Frf(1) ) / Frf(3);
zmplf_x = ( -Flf(5) -0.1189 * Flf(1) ) / Flf(3);

zmp_x = (zmprf_x * Frf(3) + zmplf_x * Flf(3))/ (Frf(3)+Flf(3));

% front edge limit = 0.12
% back edge limit = -0.055
if zmp_x < 0.12
    p1 = contact_CD(1*4+ind4);
    p2 = contact_CD(2*4+ind4);
else
    p1 = contact_AB(1*4+ind4);
    p2 = contact_AB(2*4+ind4);
end

p1rf_s = Hrf * p1;
p2rf_s = Hrf * p2;

p1lf_s = Hlf * p1;
p2lf_s = Hlf * p2;

pcont = [ p1rf_s(1:3) ; p2rf_s(1:3) ; p1lf_s(1:3) ; p2lf_s(1:3) ];

vcont = [ Jrf * dq; Jlf * dq ];

%measurement equation 

    y = [ jnt ; imu ; gyro ; pcont ; vcont ];
    z = z_in;


% Compute the Jacobian of acceleration terms(forward dynamics):
dimu = zeros(3,dof*2);
%dgyro = zeros(3,dof*2);
dgyro = [ zeros(3,dof+3),eye(3,28) ];
dpcont = zeros(12,dof*2);
dvcont = zeros(12,dof*2);

for i = 1:62
    dM   = M_in(i*dof+(1:dof),:);
    dC   = C_in(i*dof+(1:dof),:);
    dg   = g_in(i*dof+(1:dof));
    dJrf = J_in(i*30+(1*6+ind6),:);
    dJlf = J_in(i*30+(2*6+ind6),:);
    
    dHfb = H_in(i*20+(5*4+ind4),:);
    dRfb  = dHfb( 1:3, 1:3);
    
    dHrf = H_in(i*20+(1*4+ind4),:);
    dRrf = dHrf(1:3,1:3);
    dprf = Skew(dHrf(1:3,4));
    dAdrf   = [ dRrf dprf*Rrf+prf*dRrf ; zeros(3) dRrf ];
    
    dHlf = H_in(i*20+(2*4+ind4),:);
    dRlf = dHlf(1:3,1:3);
    dplf = Skew(dHlf(1:3,4));
    dAdlf   = [ dRlf dplf*Rlf+plf*dRlf ; zeros(3) dRlf ];
    
    %dTA  = TA_in(i*6+(1*6+ind6),:);
    
    df   = invM * (-dM*acc +(-dC*dq - dg + dJrf'*Adrf'*Frf + Jrf'*dAdrf'*Frf...
                                              + dJlf'*Adlf'*Flf + Jlf'*dAdlf'*Flf...
                                              - ( dJrf'*Irf* (invAdrf * gacc) + Jrf'*(-invAdrf *(dAdrf*(invAdrf * gacc))) ) ...
                                              - ( dJlf'*Ilf* (invAdlf * gacc) + Jlf'*(-invAdlf *(dAdlf*(invAdlf * gacc))) ) ));                                        
      
    dp1rf_s = dHrf*p1 ; dp2rf_s = dHrf*p2 ; dp1lf_s = dHlf*p1 ; dp2lf_s = dHlf*p2;
    dpcont(:,i) =[ dp1rf_s(1:3) ; dp2rf_s(1:3) ; dp1lf_s(1:3) ; dp2lf_s(1:3) ];
    dvcont(:,i) = [ dJrf * dq; dJlf * dq; ];

    if i > dof
        df = df + invM * (- C(:,i-31));
        dvcont(:,i) = dvcont(:,i) + [ Jrf(:,i-31); Jlf(:,i-31); ];
    end
    dimu(1:3,i) = df(1:3) + dRfb'*[0 0 9.81]';
end

djnt = [ [zeros(25,6),eye(25,25),zeros(25,31)]; [zeros(25,37),eye(25,25)] ];

% dgyro(1,35) = 1; 
% dgyro(2,36) = 1;
% dgyro(3,37) = 1;
% Measurement matrix

if zmp_x < -0.05 && zmp_x> 0.12
    C_uo = [ djnt ; dimu ; dgyro ; dpcont];
    R_uo = R_in(1:end-12,1:end-12);
    K_uo = P_*C_uo'/(C_uo*P_*C_uo'+R_uo);
    I = eye(size(P_));
    P = (I-K_uo*C_uo)*P_*(I-K_uo*C_uo)' + K_uo*R_uo*K_uo' ;
    x_out = x_in + K_uo *(z(1:end-12) - y(1:end-12));
else
    C_o = [ djnt ; dimu ; dgyro ; dpcont ; dvcont];
    R_o = R_in;
    K = P_*C_o'/(C_o*P_*C_o'+R_o);
    I = eye(size(P_));
    P = (I-K*C_o)*P_*(I-K*C_o)' + K*R_o*K' ;
    x_out = x_in + K *(z-y);
end
